simulink model "Simulation1"  (R2017b)
settings: Solver=FixedStepDiscrete  StartTime=0.0  StopTime=N/Fs  RelTol=1e-3
values from neighbouring files (symbols this model uses):
  A = 0.5*(nLev-1)    (= 0.5)    [Model3.m]
  ftest = 9e3    (= 9000)    [Model3.m]    (also in Model3_LTE.m = 2250)
  Ts = 1/Fs    (= 2.03450520833e-06)    [Model3.m]    (also in Model3_LTE.m = 1/Fs)
undefined symbols (not defined in the file or in its folder): a, b, c, g
libraries: dspsigops x16, simulink x8, dspsrcs4 x2
(part 1 of 3)
settings Model: Creator=o_cotte  LastModifiedBy=o_cotte

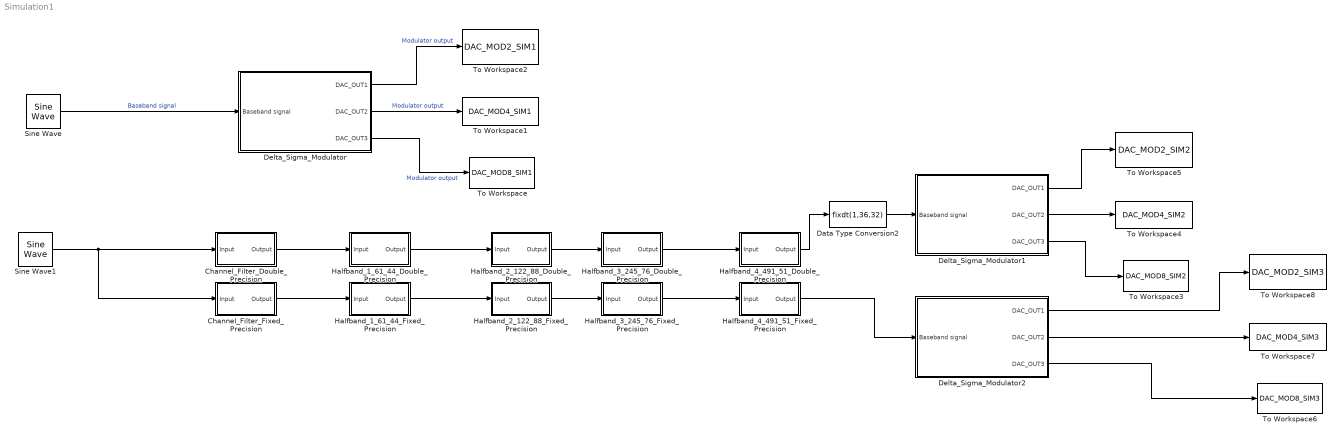
== system Simulation1 ==
  Channel_Filter_Double_Precision : Subsystem  Tag=FilterWizardSubSystem
      settings: ErrorFcn=dspFilterRealizedInBasicElemsAlgLoopErrFcnCallback
  Channel_Filter_Fixed_Precision : Subsystem  Tag=FilterWizardSubSystem
      settings: ErrorFcn=dspFilterRealizedInBasicElemsAlgLoopErrFcnCallback
  Data Type Conversion2 : DataTypeConversion  OutDataTypeStr=fixdt(1,36,32)  LockScale=on
  Delta_Sigma_Modulator : Subsystem
  Delta_Sigma_Modulator1 : Subsystem
  Delta_Sigma_Modulator2 : Subsystem
  Halfband_1_61_44_Double_Precision : Subsystem  Tag=FilterWizardSubSystem
      settings: ErrorFcn=dspFilterRealizedInBasicElemsAlgLoopErrFcnCallback
  Halfband_1_61_44_Fixed_Precision : Subsystem  Tag=FilterWizardSubSystem
      settings: ErrorFcn=dspFilterRealizedInBasicElemsAlgLoopErrFcnCallback
  Halfband_2_122_88_Double_Precision : Subsystem  Tag=FilterWizardSubSystem
      settings: ErrorFcn=dspFilterRealizedInBasicElemsAlgLoopErrFcnCallback
  Halfband_2_122_88_Fixed_Precision : Subsystem  Tag=FilterWizardSubSystem
      settings: ErrorFcn=dspFilterRealizedInBasicElemsAlgLoopErrFcnCallback
  Halfband_3_245_76_Double_Precision : Subsystem  Tag=FilterWizardSubSystem
      settings: ErrorFcn=dspFilterRealizedInBasicElemsAlgLoopErrFcnCallback
  Halfband_3_245_76_Fixed_Precision : Subsystem  Tag=FilterWizardSubSystem
      settings: ErrorFcn=dspFilterRealizedInBasicElemsAlgLoopErrFcnCallback
  Halfband_4_491_51_Double_Precision : Subsystem  Tag=FilterWizardSubSystem
      settings: ErrorFcn=dspFilterRealizedInBasicElemsAlgLoopErrFcnCallback
  Halfband_4_491_51_Fixed_Precision : Subsystem  Tag=FilterWizardSubSystem
      settings: ErrorFcn=dspFilterRealizedInBasicElemsAlgLoopErrFcnCallback
  Sine Wave : dspsrcs4/Sine Wave  Amplitude=0.77  Frequency=ftest  Phase=0  SampleMode=Discrete  OutComplex=Real  CompMethod=Trigonometric fcn  TableSize=Speed  SampleTime=Ts  SamplesPerFrame=1  ResetState=Restart at time zero  OutputFrames=on  dataType=double  wordLen=16  udDataType=sfix(16)  fracBitsMode=Best precision  numFracBits=15  OutDataTypeStr=double  LastOutDataTypeStr=double
  Sine Wave1 : dspsrcs4/Sine Wave  Amplitude=A  Frequency=ftest  Phase=0  SampleMode=Discrete  OutComplex=Real  CompMethod=Trigonometric fcn  TableSize=Speed  SampleTime=1/30.72e3  SamplesPerFrame=1  ResetState=Restart at time zero  OutputFrames=on  dataType=double  wordLen=16  udDataType=sfix(16)  fracBitsMode=Best precision  numFracBits=15  OutDataTypeStr=double  LastOutDataTypeStr=double
  To Workspace : ToWorkspace  VariableName=DAC_MOD8_SIM1  SampleTime=-1
  To Workspace1 : ToWorkspace  VariableName=DAC_MOD4_SIM1  SampleTime=-1
  To Workspace2 : ToWorkspace  VariableName=DAC_MOD2_SIM1  SampleTime=-1
  To Workspace3 : ToWorkspace  VariableName=DAC_MOD8_SIM2  SampleTime=-1
  To Workspace4 : ToWorkspace  VariableName=DAC_MOD4_SIM2  SampleTime=-1
  To Workspace5 : ToWorkspace  VariableName=DAC_MOD2_SIM2  SampleTime=-1
  To Workspace6 : ToWorkspace  VariableName=DAC_MOD8_SIM3  SampleTime=-1
  To Workspace7 : ToWorkspace  VariableName=DAC_MOD4_SIM3  SampleTime=-1
  To Workspace8 : ToWorkspace  VariableName=DAC_MOD2_SIM3  SampleTime=-1
  wires:
  Sine Wave/1 -> Delta_Sigma_Modulator/1(Baseband signal)  "Baseband signal"
  Delta_Sigma_Modulator/3(DAC_OUT3) -> To Workspace/1  "Modulator output"
  Delta_Sigma_Modulator/2(DAC_OUT2) -> To Workspace1/1  "Modulator output"
  Delta_Sigma_Modulator/1(DAC_OUT1) -> To Workspace2/1  "Modulator output"
  Channel_Filter_Double_Precision/1(Output) -> Halfband_1_61_44_Double_Precision/1(Input)
  Halfband_1_61_44_Double_Precision/1(Output) -> Halfband_2_122_88_Double_Precision/1(Input)
  Halfband_2_122_88_Double_Precision/1(Output) -> Halfband_3_245_76_Double_Precision/1(Input)
  Halfband_3_245_76_Double_Precision/1(Output) -> Halfband_4_491_51_Double_Precision/1(Input)
  Halfband_3_245_76_Fixed_Precision/1(Output) -> Halfband_4_491_51_Fixed_Precision/1(Input)
  Halfband_2_122_88_Fixed_Precision/1(Output) -> Halfband_3_245_76_Fixed_Precision/1(Input)
  Halfband_1_61_44_Fixed_Precision/1(Output) -> Halfband_2_122_88_Fixed_Precision/1(Input)
  Channel_Filter_Fixed_Precision/1(Output) -> Halfband_1_61_44_Fixed_Precision/1(Input)
  Sine Wave1/1 -> Channel_Filter_Fixed_Precision/1(Input), Channel_Filter_Double_Precision/1(Input)
  Halfband_4_491_51_Fixed_Precision/1(Output) -> Delta_Sigma_Modulator2/1(Baseband signal)
  Delta_Sigma_Modulator1/2(DAC_OUT2) -> To Workspace4/1
  Delta_Sigma_Modulator1/3(DAC_OUT3) -> To Workspace3/1
  Delta_Sigma_Modulator1/1(DAC_OUT1) -> To Workspace5/1
  Delta_Sigma_Modulator2/2(DAC_OUT2) -> To Workspace7/1
  Delta_Sigma_Modulator2/1(DAC_OUT1) -> To Workspace8/1
  Delta_Sigma_Modulator2/3(DAC_OUT3) -> To Workspace6/1
  Data Type Conversion2/1 -> Delta_Sigma_Modulator1/1(Baseband signal)
  Halfband_4_491_51_Double_Precision/1(Output) -> Data Type Conversion2/1

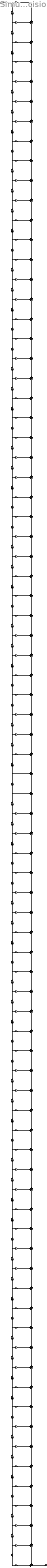
== system Simulation1/Channel_Filter_Double_Precision ==
  Input : Inport
  BodyDelay{2..80} (79 alike) : Delay  DelayLength=1  InitialCondition=0
  BodyLSum{2..80} (79 alike) : Sum  Inputs=++|  RndMeth=Nearest  SaturateOnIntegerOverflow=on  OutDataTypeStr=Inherit: Same as first input
  b(1) : Gain  Gain=0.00196720306212561482  ParamDataTypeStr=double  RndMeth=Nearest  SaturateOnIntegerOverflow=on  OutDataTypeStr=Inherit: Same as input
  b(10) : Gain  Gain=0.00124990544593627895  ParamDataTypeStr=double  RndMeth=Nearest  SaturateOnIntegerOverflow=on  OutDataTypeStr=Inherit: Same as input
  b(11) : Gain  Gain=0.00637795842127835896  ParamDataTypeStr=double  RndMeth=Nearest  SaturateOnIntegerOverflow=on  OutDataTypeStr=Inherit: Same as input
  b(12) : Gain  Gain=-0.00686348731071946636  ParamDataTypeStr=double  RndMeth=Nearest  SaturateOnIntegerOverflow=on  OutDataTypeStr=Inherit: Same as input
  b(13) : Gain  Gain=-0.00221497240802292442  ParamDataTypeStr=double  RndMeth=Nearest  SaturateOnIntegerOverflow=on  OutDataTypeStr=Inherit: Same as input
  b(14) : Gain  Gain=0.0103098487689475479  ParamDataTypeStr=double  RndMeth=Nearest  SaturateOnIntegerOverflow=on  OutDataTypeStr=Inherit: Same as input
  b(15) : Gain  Gain=-0.00579957522561930575  ParamDataTypeStr=double  RndMeth=Nearest  SaturateOnIntegerOverflow=on  OutDataTypeStr=Inherit: Same as input
  b(16) : Gain  Gain=-0.00783937474606764828  ParamDataTypeStr=double  RndMeth=Nearest  SaturateOnIntegerOverflow=on  OutDataTypeStr=Inherit: Same as input
  b(17) : Gain  Gain=0.0135158399775277549  ParamDataTypeStr=double  RndMeth=Nearest  SaturateOnIntegerOverflow=on  OutDataTypeStr=Inherit: Same as input
  b(18) : Gain  Gain=-0.00155602281125578911  ParamDataTypeStr=double  RndMeth=Nearest  SaturateOnIntegerOverflow=on  OutDataTypeStr=Inherit: Same as input
  b(19) : Gain  Gain=-0.0151258138642529176  ParamDataTypeStr=double  RndMeth=Nearest  SaturateOnIntegerOverflow=on  OutDataTypeStr=Inherit: Same as input
  b(2) : Gain  Gain=0.00149425216106443691  ParamDataTypeStr=double  RndMeth=Nearest  SaturateOnIntegerOverflow=on  OutDataTypeStr=Inherit: Same as input
  b(20) : Gain  Gain=0.0142568491821450007  ParamDataTypeStr=double  RndMeth=Nearest  SaturateOnIntegerOverflow=on  OutDataTypeStr=Inherit: Same as input
  b(21) : Gain  Gain=0.00665092392134642753  ParamDataTypeStr=double  RndMeth=Nearest  SaturateOnIntegerOverflow=on  OutDataTypeStr=Inherit: Same as input
  b(22) : Gain  Gain=-0.0226731257471077807  ParamDataTypeStr=double  RndMeth=Nearest  SaturateOnIntegerOverflow=on  OutDataTypeStr=Inherit: Same as input
  b(23) : Gain  Gain=0.0104679129061562917  ParamDataTypeStr=double  RndMeth=Nearest  SaturateOnIntegerOverflow=on  OutDataTypeStr=Inherit: Same as input
  b(24) : Gain  Gain=0.018904809782294061  ParamDataTypeStr=double  RndMeth=Nearest  SaturateOnIntegerOverflow=on  OutDataTypeStr=Inherit: Same as input
  b(25) : Gain  Gain=-0.0281519456111425509  ParamDataTypeStr=double  RndMeth=Nearest  SaturateOnIntegerOverflow=on  OutDataTypeStr=Inherit: Same as input
  b(26) : Gain  Gain=3.77195008409268937e-05  ParamDataTypeStr=double  RndMeth=Nearest  SaturateOnIntegerOverflow=on  OutDataTypeStr=Inherit: Same as input
  b(27) : Gain  Gain=0.0343690574379760388  ParamDataTypeStr=double  RndMeth=Nearest  SaturateOnIntegerOverflow=on  OutDataTypeStr=Inherit: Same as input
  b(28) : Gain  Gain=-0.0283201893723893684  ParamDataTypeStr=double  RndMeth=Nearest  SaturateOnIntegerOverflow=on  OutDataTypeStr=Inherit: Same as input
  b(29) : Gain  Gain=-0.0191525533345231584  ParamDataTypeStr=double  RndMeth=Nearest  SaturateOnIntegerOverflow=on  OutDataTypeStr=Inherit: Same as input
  b(3) : Gain  Gain=-0.00400293320810243911  ParamDataTypeStr=double  RndMeth=Nearest  SaturateOnIntegerOverflow=on  OutDataTypeStr=Inherit: Same as input
  b(30) : Gain  Gain=0.0512858826615412086  ParamDataTypeStr=double  RndMeth=Nearest  SaturateOnIntegerOverflow=on  OutDataTypeStr=Inherit: Same as input
  b(31) : Gain  Gain=-0.0186277130508248137  ParamDataTypeStr=double  RndMeth=Nearest  SaturateOnIntegerOverflow=on  OutDataTypeStr=Inherit: Same as input
  b(32) : Gain  Gain=-0.0502110306645960694  ParamDataTypeStr=double  RndMeth=Nearest  SaturateOnIntegerOverflow=on  OutDataTypeStr=Inherit: Same as input
  b(33) : Gain  Gain=0.0672661641118006554  ParamDataTypeStr=double  RndMeth=Nearest  SaturateOnIntegerOverflow=on  OutDataTypeStr=Inherit: Same as input
  b(34) : Gain  Gain=0.00945698178191303231  ParamDataTypeStr=double  RndMeth=Nearest  SaturateOnIntegerOverflow=on  OutDataTypeStr=Inherit: Same as input
  b(35) : Gain  Gain=-0.102591535984214791  ParamDataTypeStr=double  RndMeth=Nearest  SaturateOnIntegerOverflow=on  OutDataTypeStr=Inherit: Same as input
  b(36) : Gain  Gain=0.0797527182394069389  ParamDataTypeStr=double  RndMeth=Nearest  SaturateOnIntegerOverflow=on  OutDataTypeStr=Inherit: Same as input
  b(37) : Gain  Gain=0.0877414496207477579  ParamDataTypeStr=double  RndMeth=Nearest  SaturateOnIntegerOverflow=on  OutDataTypeStr=Inherit: Same as input
  b(38) : Gain  Gain=-0.237055871068311774  ParamDataTypeStr=double  RndMeth=Nearest  SaturateOnIntegerOverflow=on  OutDataTypeStr=Inherit: Same as input
  b(39) : Gain  Gain=0.0866069815926385905  ParamDataTypeStr=double  RndMeth=Nearest  SaturateOnIntegerOverflow=on  OutDataTypeStr=Inherit: Same as input
  b(4) : Gain  Gain=0.00390100375479263085  ParamDataTypeStr=double  RndMeth=Nearest  SaturateOnIntegerOverflow=on  OutDataTypeStr=Inherit: Same as input
  b(42) : Gain  Gain=0.0866069815926385905  ParamDataTypeStr=double  RndMeth=Nearest  SaturateOnIntegerOverflow=on  OutDataTypeStr=Inherit: Same as input
  b(43) : Gain  Gain=-0.237055871068311774  ParamDataTypeStr=double  RndMeth=Nearest  SaturateOnIntegerOverflow=on  OutDataTypeStr=Inherit: Same as input
  b(44) : Gain  Gain=0.0877414496207477579  ParamDataTypeStr=double  RndMeth=Nearest  SaturateOnIntegerOverflow=on  OutDataTypeStr=Inherit: Same as input
  b(45) : Gain  Gain=0.0797527182394069389  ParamDataTypeStr=double  RndMeth=Nearest  SaturateOnIntegerOverflow=on  OutDataTypeStr=Inherit: Same as input
  b(46) : Gain  Gain=-0.102591535984214791  ParamDataTypeStr=double  RndMeth=Nearest  SaturateOnIntegerOverflow=on  OutDataTypeStr=Inherit: Same as input
  b(47) : Gain  Gain=0.00945698178191303231  ParamDataTypeStr=double  RndMeth=Nearest  SaturateOnIntegerOverflow=on  OutDataTypeStr=Inherit: Same as input
  b(48) : Gain  Gain=0.0672661641118006554  ParamDataTypeStr=double  RndMeth=Nearest  SaturateOnIntegerOverflow=on  OutDataTypeStr=Inherit: Same as input
  b(49) : Gain  Gain=-0.0502110306645960694  ParamDataTypeStr=double  RndMeth=Nearest  SaturateOnIntegerOverflow=on  OutDataTypeStr=Inherit: Same as input
  b(5) : Gain  Gain=-2.89147778793418149e-07  ParamDataTypeStr=double  RndMeth=Nearest  SaturateOnIntegerOverflow=on  OutDataTypeStr=Inherit: Same as input
  b(50) : Gain  Gain=-0.0186277130508248137  ParamDataTypeStr=double  RndMeth=Nearest  SaturateOnIntegerOverflow=on  OutDataTypeStr=Inherit: Same as input
  b(51) : Gain  Gain=0.0512858826615412086  ParamDataTypeStr=double  RndMeth=Nearest  SaturateOnIntegerOverflow=on  OutDataTypeStr=Inherit: Same as input
  b(52) : Gain  Gain=-0.0191525533345231584  ParamDataTypeStr=double  RndMeth=Nearest  SaturateOnIntegerOverflow=on  OutDataTypeStr=Inherit: Same as input
  b(53) : Gain  Gain=-0.0283201893723893684  ParamDataTypeStr=double  RndMeth=Nearest  SaturateOnIntegerOverflow=on  OutDataTypeStr=Inherit: Same as input
  b(54) : Gain  Gain=0.0343690574379760388  ParamDataTypeStr=double  RndMeth=Nearest  SaturateOnIntegerOverflow=on  OutDataTypeStr=Inherit: Same as input
  b(55) : Gain  Gain=3.77195008409268937e-05  ParamDataTypeStr=double  RndMeth=Nearest  SaturateOnIntegerOverflow=on  OutDataTypeStr=Inherit: Same as input
  b(56) : Gain  Gain=-0.0281519456111425509  ParamDataTypeStr=double  RndMeth=Nearest  SaturateOnIntegerOverflow=on  OutDataTypeStr=Inherit: Same as input
  b(57) : Gain  Gain=0.018904809782294061  ParamDataTypeStr=double  RndMeth=Nearest  SaturateOnIntegerOverflow=on  OutDataTypeStr=Inherit: Same as input
  b(58) : Gain  Gain=0.0104679129061562917  ParamDataTypeStr=double  RndMeth=Nearest  SaturateOnIntegerOverflow=on  OutDataTypeStr=Inherit: Same as input
  b(59) : Gain  Gain=-0.0226731257471077807  ParamDataTypeStr=double  RndMeth=Nearest  SaturateOnIntegerOverflow=on  OutDataTypeStr=Inherit: Same as input
  b(6) : Gain  Gain=-0.00382987035567847927  ParamDataTypeStr=double  RndMeth=Nearest  SaturateOnIntegerOverflow=on  OutDataTypeStr=Inherit: Same as input
  b(60) : Gain  Gain=0.00665092392134642753  ParamDataTypeStr=double  RndMeth=Nearest  SaturateOnIntegerOverflow=on  OutDataTypeStr=Inherit: Same as input
  b(61) : Gain  Gain=0.0142568491821450007  ParamDataTypeStr=double  RndMeth=Nearest  SaturateOnIntegerOverflow=on  OutDataTypeStr=Inherit: Same as input
  b(62) : Gain  Gain=-0.0151258138642529176  ParamDataTypeStr=double  RndMeth=Nearest  SaturateOnIntegerOverflow=on  OutDataTypeStr=Inherit: Same as input
  b(63) : Gain  Gain=-0.00155602281125578911  ParamDataTypeStr=double  RndMeth=Nearest  SaturateOnIntegerOverflow=on  OutDataTypeStr=Inherit: Same as input
  b(64) : Gain  Gain=0.0135158399775277549  ParamDataTypeStr=double  RndMeth=Nearest  SaturateOnIntegerOverflow=on  OutDataTypeStr=Inherit: Same as input
  b(65) : Gain  Gain=-0.00783937474606764828  ParamDataTypeStr=double  RndMeth=Nearest  SaturateOnIntegerOverflow=on  OutDataTypeStr=Inherit: Same as input
  b(66) : Gain  Gain=-0.00579957522561930575  ParamDataTypeStr=double  RndMeth=Nearest  SaturateOnIntegerOverflow=on  OutDataTypeStr=Inherit: Same as input
  b(67) : Gain  Gain=0.0103098487689475479  ParamDataTypeStr=double  RndMeth=Nearest  SaturateOnIntegerOverflow=on  OutDataTypeStr=Inherit: Same as input
  b(68) : Gain  Gain=-0.00221497240802292442  ParamDataTypeStr=double  RndMeth=Nearest  SaturateOnIntegerOverflow=on  OutDataTypeStr=Inherit: Same as input
  b(69) : Gain  Gain=-0.00686348731071946636  ParamDataTypeStr=double  RndMeth=Nearest  SaturateOnIntegerOverflow=on  OutDataTypeStr=Inherit: Same as input
  b(7) : Gain  Gain=0.00259524746093026722  ParamDataTypeStr=double  RndMeth=Nearest  SaturateOnIntegerOverflow=on  OutDataTypeStr=Inherit: Same as input
  b(70) : Gain  Gain=0.00637795842127835896  ParamDataTypeStr=double  RndMeth=Nearest  SaturateOnIntegerOverflow=on  OutDataTypeStr=Inherit: Same as input
  b(71) : Gain  Gain=0.00124990544593627895  ParamDataTypeStr=double  RndMeth=Nearest  SaturateOnIntegerOverflow=on  OutDataTypeStr=Inherit: Same as input
  b(72) : Gain  Gain=-0.00593452115673513431  ParamDataTypeStr=double  RndMeth=Nearest  SaturateOnIntegerOverflow=on  OutDataTypeStr=Inherit: Same as input
  b(73) : Gain  Gain=0.00299398664123881825  ParamDataTypeStr=double  RndMeth=Nearest  SaturateOnIntegerOverflow=on  OutDataTypeStr=Inherit: Same as input
  b(74) : Gain  Gain=0.00259524746093026722  ParamDataTypeStr=double  RndMeth=Nearest  SaturateOnIntegerOverflow=on  OutDataTypeStr=Inherit: Same as input
  b(75) : Gain  Gain=-0.00382987035567847927  ParamDataTypeStr=double  RndMeth=Nearest  SaturateOnIntegerOverflow=on  OutDataTypeStr=Inherit: Same as input
  b(76) : Gain  Gain=-2.89147778793418149e-07  ParamDataTypeStr=double  RndMeth=Nearest  SaturateOnIntegerOverflow=on  OutDataTypeStr=Inherit: Same as input
  b(77) : Gain  Gain=0.00390100375479263085  ParamDataTypeStr=double  RndMeth=Nearest  SaturateOnIntegerOverflow=on  OutDataTypeStr=Inherit: Same as input
  b(78) : Gain  Gain=-0.00400293320810243911  ParamDataTypeStr=double  RndMeth=Nearest  SaturateOnIntegerOverflow=on  OutDataTypeStr=Inherit: Same as input
  b(79) : Gain  Gain=0.00149425216106443691  ParamDataTypeStr=double  RndMeth=Nearest  SaturateOnIntegerOverflow=on  OutDataTypeStr=Inherit: Same as input
  b(8) : Gain  Gain=0.00299398664123881825  ParamDataTypeStr=double  RndMeth=Nearest  SaturateOnIntegerOverflow=on  OutDataTypeStr=Inherit: Same as input
  b(80) : Gain  Gain=0.00196720306212561482  ParamDataTypeStr=double  RndMeth=Nearest  SaturateOnIntegerOverflow=on  OutDataTypeStr=Inherit: Same as input
  b(9) : Gain  Gain=-0.00593452115673513431  ParamDataTypeStr=double  RndMeth=Nearest  SaturateOnIntegerOverflow=on  OutDataTypeStr=Inherit: Same as input
  Output : Outport
  wires:
  Input/1 -> b(1)/1, BodyDelay2/1
  b(1)/1 -> BodyLSum2/2
  BodyDelay2/1 -> b(2)/1, BodyDelay3/1
  b(2)/1 -> BodyLSum2/1
  BodyLSum2/1 -> BodyLSum3/2
  BodyDelay3/1 -> b(3)/1, BodyDelay4/1
  b(3)/1 -> BodyLSum3/1
  BodyLSum3/1 -> BodyLSum4/2
  BodyDelay4/1 -> b(4)/1, BodyDelay5/1
  b(4)/1 -> BodyLSum4/1
  BodyLSum4/1 -> BodyLSum5/2
  BodyDelay5/1 -> b(5)/1, BodyDelay6/1
  b(5)/1 -> BodyLSum5/1
  BodyLSum5/1 -> BodyLSum6/2
  BodyDelay6/1 -> b(6)/1, BodyDelay7/1
  b(6)/1 -> BodyLSum6/1
  BodyLSum6/1 -> BodyLSum7/2
  BodyDelay7/1 -> b(7)/1, BodyDelay8/1
  b(7)/1 -> BodyLSum7/1
  BodyLSum7/1 -> BodyLSum8/2
  BodyDelay8/1 -> b(8)/1, BodyDelay9/1
  b(8)/1 -> BodyLSum8/1
  BodyLSum8/1 -> BodyLSum9/2
  BodyDelay9/1 -> b(9)/1, BodyDelay10/1
  b(9)/1 -> BodyLSum9/1
  BodyLSum9/1 -> BodyLSum10/2
  BodyDelay10/1 -> b(10)/1, BodyDelay11/1
  b(10)/1 -> BodyLSum10/1
  BodyLSum10/1 -> BodyLSum11/2
  BodyDelay11/1 -> b(11)/1, BodyDelay12/1
  b(11)/1 -> BodyLSum11/1
  BodyLSum11/1 -> BodyLSum12/2
  BodyDelay12/1 -> b(12)/1, BodyDelay13/1
  b(12)/1 -> BodyLSum12/1
  BodyLSum12/1 -> BodyLSum13/2
  BodyDelay13/1 -> b(13)/1, BodyDelay14/1
  b(13)/1 -> BodyLSum13/1
  BodyLSum13/1 -> BodyLSum14/2
  BodyDelay14/1 -> b(14)/1, BodyDelay15/1
  b(14)/1 -> BodyLSum14/1
  BodyLSum14/1 -> BodyLSum15/2
  BodyDelay15/1 -> b(15)/1, BodyDelay16/1
  b(15)/1 -> BodyLSum15/1
  BodyLSum15/1 -> BodyLSum16/2
  BodyDelay16/1 -> b(16)/1, BodyDelay17/1
  b(16)/1 -> BodyLSum16/1
  BodyLSum16/1 -> BodyLSum17/2
  BodyDelay17/1 -> b(17)/1, BodyDelay18/1
  b(17)/1 -> BodyLSum17/1
  BodyLSum17/1 -> BodyLSum18/2
  BodyDelay18/1 -> b(18)/1, BodyDelay19/1
  b(18)/1 -> BodyLSum18/1
  BodyLSum18/1 -> BodyLSum19/2
  BodyDelay19/1 -> b(19)/1, BodyDelay20/1
  b(19)/1 -> BodyLSum19/1
  BodyLSum19/1 -> BodyLSum20/2
  BodyDelay20/1 -> b(20)/1, BodyDelay21/1
  b(20)/1 -> BodyLSum20/1
  BodyLSum20/1 -> BodyLSum21/2
  BodyDelay21/1 -> b(21)/1, BodyDelay22/1
  b(21)/1 -> BodyLSum21/1
  BodyLSum21/1 -> BodyLSum22/2
  BodyDelay22/1 -> b(22)/1, BodyDelay23/1
  b(22)/1 -> BodyLSum22/1
  BodyLSum22/1 -> BodyLSum23/2
  BodyDelay23/1 -> b(23)/1, BodyDelay24/1
  b(23)/1 -> BodyLSum23/1
  BodyLSum23/1 -> BodyLSum24/2
  BodyDelay24/1 -> b(24)/1, BodyDelay25/1
  b(24)/1 -> BodyLSum24/1
  BodyLSum24/1 -> BodyLSum25/2
  BodyDelay25/1 -> b(25)/1, BodyDelay26/1
  b(25)/1 -> BodyLSum25/1
  BodyLSum25/1 -> BodyLSum26/2
  BodyDelay26/1 -> b(26)/1, BodyDelay27/1
  b(26)/1 -> BodyLSum26/1
  BodyLSum26/1 -> BodyLSum27/2
  BodyDelay27/1 -> b(27)/1, BodyDelay28/1
  b(27)/1 -> BodyLSum27/1
  BodyLSum27/1 -> BodyLSum28/2
  BodyDelay28/1 -> b(28)/1, BodyDelay29/1
  b(28)/1 -> BodyLSum28/1
  BodyLSum28/1 -> BodyLSum29/2
  BodyDelay29/1 -> b(29)/1, BodyDelay30/1
  b(29)/1 -> BodyLSum29/1
  BodyLSum29/1 -> BodyLSum30/2
  BodyDelay30/1 -> b(30)/1, BodyDelay31/1
  b(30)/1 -> BodyLSum30/1
  BodyLSum30/1 -> BodyLSum31/2
  BodyDelay31/1 -> b(31)/1, BodyDelay32/1
  b(31)/1 -> BodyLSum31/1
  BodyLSum31/1 -> BodyLSum32/2
  BodyDelay32/1 -> b(32)/1, BodyDelay33/1
  b(32)/1 -> BodyLSum32/1
  BodyLSum32/1 -> BodyLSum33/2
  BodyDelay33/1 -> b(33)/1, BodyDelay34/1
  b(33)/1 -> BodyLSum33/1
  BodyLSum33/1 -> BodyLSum34/2
  BodyDelay34/1 -> b(34)/1, BodyDelay35/1
  b(34)/1 -> BodyLSum34/1
  BodyLSum34/1 -> BodyLSum35/2
  BodyDelay35/1 -> b(35)/1, BodyDelay36/1
  b(35)/1 -> BodyLSum35/1
  BodyLSum35/1 -> BodyLSum36/2
  BodyDelay36/1 -> b(36)/1, BodyDelay37/1
  b(36)/1 -> BodyLSum36/1
  BodyLSum36/1 -> BodyLSum37/2
  BodyDelay37/1 -> b(37)/1, BodyDelay38/1
  b(37)/1 -> BodyLSum37/1
  BodyLSum37/1 -> BodyLSum38/2
  BodyDelay38/1 -> b(38)/1, BodyDelay39/1
  b(38)/1 -> BodyLSum38/1
  BodyLSum38/1 -> BodyLSum39/2
  BodyDelay39/1 -> b(39)/1, BodyDelay40/1
  b(39)/1 -> BodyLSum39/1
  BodyLSum39/1 -> BodyLSum40/2
  BodyDelay40/1 -> BodyLSum40/1, BodyDelay41/1
  BodyLSum40/1 -> BodyLSum41/2
  BodyDelay41/1 -> BodyLSum41/1, BodyDelay42/1
  BodyLSum41/1 -> BodyLSum42/2
  BodyDelay42/1 -> b(42)/1, BodyDelay43/1
  b(42)/1 -> BodyLSum42/1
  BodyLSum42/1 -> BodyLSum43/2
  BodyDelay43/1 -> b(43)/1, BodyDelay44/1
  b(43)/1 -> BodyLSum43/1
  BodyLSum43/1 -> BodyLSum44/2
  BodyDelay44/1 -> b(44)/1, BodyDelay45/1
  b(44)/1 -> BodyLSum44/1
  BodyLSum44/1 -> BodyLSum45/2
  BodyDelay45/1 -> b(45)/1, BodyDelay46/1
  b(45)/1 -> BodyLSum45/1
  BodyLSum45/1 -> BodyLSum46/2
  BodyDelay46/1 -> b(46)/1, BodyDelay47/1
  b(46)/1 -> BodyLSum46/1
  BodyLSum46/1 -> BodyLSum47/2
  BodyDelay47/1 -> b(47)/1, BodyDelay48/1
  b(47)/1 -> BodyLSum47/1
  BodyLSum47/1 -> BodyLSum48/2
  BodyDelay48/1 -> b(48)/1, BodyDelay49/1
  b(48)/1 -> BodyLSum48/1
  BodyLSum48/1 -> BodyLSum49/2
  BodyDelay49/1 -> b(49)/1, BodyDelay50/1
  b(49)/1 -> BodyLSum49/1
  BodyLSum49/1 -> BodyLSum50/2
  BodyDelay50/1 -> b(50)/1, BodyDelay51/1
  b(50)/1 -> BodyLSum50/1
  BodyLSum50/1 -> BodyLSum51/2
  BodyDelay51/1 -> b(51)/1, BodyDelay52/1
  b(51)/1 -> BodyLSum51/1
  BodyLSum51/1 -> BodyLSum52/2
  BodyDelay52/1 -> b(52)/1, BodyDelay53/1
  b(52)/1 -> BodyLSum52/1
  BodyLSum52/1 -> BodyLSum53/2
  BodyDelay53/1 -> b(53)/1, BodyDelay54/1
  b(53)/1 -> BodyLSum53/1
  BodyLSum53/1 -> BodyLSum54/2
  BodyDelay54/1 -> b(54)/1, BodyDelay55/1
  b(54)/1 -> BodyLSum54/1
  BodyLSum54/1 -> BodyLSum55/2
  BodyDelay55/1 -> b(55)/1, BodyDelay56/1
  b(55)/1 -> BodyLSum55/1
  BodyLSum55/1 -> BodyLSum56/2
  BodyDelay56/1 -> b(56)/1, BodyDelay57/1
  b(56)/1 -> BodyLSum56/1
  BodyLSum56/1 -> BodyLSum57/2
  BodyDelay57/1 -> b(57)/1, BodyDelay58/1
  b(57)/1 -> BodyLSum57/1
  BodyLSum57/1 -> BodyLSum58/2
  BodyDelay58/1 -> b(58)/1, BodyDelay59/1
  b(58)/1 -> BodyLSum58/1
  BodyLSum58/1 -> BodyLSum59/2
  BodyDelay59/1 -> b(59)/1, BodyDelay60/1
  b(59)/1 -> BodyLSum59/1
  BodyLSum59/1 -> BodyLSum60/2
  BodyDelay60/1 -> b(60)/1, BodyDelay61/1
  b(60)/1 -> BodyLSum60/1
  BodyLSum60/1 -> BodyLSum61/2
  BodyDelay61/1 -> b(61)/1, BodyDelay62/1
  b(61)/1 -> BodyLSum61/1
  BodyLSum61/1 -> BodyLSum62/2
  BodyDelay62/1 -> b(62)/1, BodyDelay63/1
  b(62)/1 -> BodyLSum62/1
  BodyLSum62/1 -> BodyLSum63/2
  BodyDelay63/1 -> b(63)/1, BodyDelay64/1
  b(63)/1 -> BodyLSum63/1
  BodyLSum63/1 -> BodyLSum64/2
  BodyDelay64/1 -> b(64)/1, BodyDelay65/1
  b(64)/1 -> BodyLSum64/1
  BodyLSum64/1 -> BodyLSum65/2
  BodyDelay65/1 -> b(65)/1, BodyDelay66/1
  b(65)/1 -> BodyLSum65/1
  BodyLSum65/1 -> BodyLSum66/2
  BodyDelay66/1 -> b(66)/1, BodyDelay67/1
  b(66)/1 -> BodyLSum66/1
  BodyLSum66/1 -> BodyLSum67/2
  BodyDelay67/1 -> b(67)/1, BodyDelay68/1
  b(67)/1 -> BodyLSum67/1
  BodyLSum67/1 -> BodyLSum68/2
  BodyDelay68/1 -> b(68)/1, BodyDelay69/1
  b(68)/1 -> BodyLSum68/1
  BodyLSum68/1 -> BodyLSum69/2
  BodyDelay69/1 -> b(69)/1, BodyDelay70/1
  b(69)/1 -> BodyLSum69/1
  BodyLSum69/1 -> BodyLSum70/2
  BodyDelay70/1 -> b(70)/1, BodyDelay71/1
  b(70)/1 -> BodyLSum70/1
  BodyLSum70/1 -> BodyLSum71/2
  BodyDelay71/1 -> b(71)/1, BodyDelay72/1
  b(71)/1 -> BodyLSum71/1
  BodyLSum71/1 -> BodyLSum72/2
  BodyDelay72/1 -> b(72)/1, BodyDelay73/1
  b(72)/1 -> BodyLSum72/1
  BodyLSum72/1 -> BodyLSum73/2
  BodyDelay73/1 -> b(73)/1, BodyDelay74/1
  b(73)/1 -> BodyLSum73/1
  BodyLSum73/1 -> BodyLSum74/2
  BodyDelay74/1 -> b(74)/1, BodyDelay75/1
  b(74)/1 -> BodyLSum74/1
  BodyLSum74/1 -> BodyLSum75/2
  BodyDelay75/1 -> b(75)/1, BodyDelay76/1
  b(75)/1 -> BodyLSum75/1
  BodyLSum75/1 -> BodyLSum76/2
  BodyDelay76/1 -> b(76)/1, BodyDelay77/1
  b(76)/1 -> BodyLSum76/1
  BodyLSum76/1 -> BodyLSum77/2
  BodyDelay77/1 -> b(77)/1, BodyDelay78/1
  b(77)/1 -> BodyLSum77/1
  BodyLSum77/1 -> BodyLSum78/2
  BodyDelay78/1 -> b(78)/1, BodyDelay79/1
  b(78)/1 -> BodyLSum78/1
  BodyLSum78/1 -> BodyLSum79/2
  BodyDelay79/1 -> b(79)/1, BodyDelay80/1
  b(79)/1 -> BodyLSum79/1
  BodyLSum79/1 -> BodyLSum80/1
  BodyDelay80/1 -> b(80)/1
  b(80)/1 -> BodyLSum80/2
  BodyLSum80/1 -> Output/1

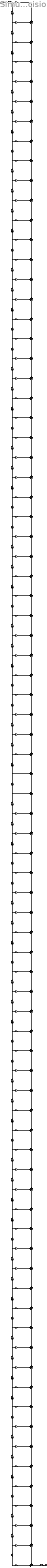
== system Simulation1/Channel_Filter_Fixed_Precision ==
  Input : Inport
  BodyDelay{2..80} (79 alike) : Delay  DelayLength=1  InitialCondition=0
  BodyLSum{2..80} (79 alike) : Sum  Inputs=++|  AccumDataTypeStr=fixdt(1,71,66)  OutDataTypeStr=fixdt(1,36,32)  SaturateOnIntegerOverflow=on
  ConvertIn : DataTypeConversion  OutDataTypeStr=fixdt(1,34,32)  RndMeth=Nearest  SaturateOnIntegerOverflow=on
  ConvertOut : DataTypeConversion  OutDataTypeStr=fixdt(1,34,30)  SaturateOnIntegerOverflow=on
  b(1) : Gain  Gain=0.00196720306212561482  ParamDataTypeStr=fixdt(1,36,34)  OutDataTypeStr=fixdt(1,36,32)  SaturateOnIntegerOverflow=on
  b(10) : Gain  Gain=0.00124990544593627895  ParamDataTypeStr=fixdt(1,36,34)  OutDataTypeStr=fixdt(1,36,32)  SaturateOnIntegerOverflow=on
  b(11) : Gain  Gain=0.00637795842127835896  ParamDataTypeStr=fixdt(1,36,34)  OutDataTypeStr=fixdt(1,36,32)  SaturateOnIntegerOverflow=on
  b(12) : Gain  Gain=-0.00686348731071946636  ParamDataTypeStr=fixdt(1,36,34)  OutDataTypeStr=fixdt(1,36,32)  SaturateOnIntegerOverflow=on
  b(13) : Gain  Gain=-0.00221497240802292442  ParamDataTypeStr=fixdt(1,36,34)  OutDataTypeStr=fixdt(1,36,32)  SaturateOnIntegerOverflow=on
  b(14) : Gain  Gain=0.0103098487689475479  ParamDataTypeStr=fixdt(1,36,34)  OutDataTypeStr=fixdt(1,36,32)  SaturateOnIntegerOverflow=on
  b(15) : Gain  Gain=-0.00579957522561930575  ParamDataTypeStr=fixdt(1,36,34)  OutDataTypeStr=fixdt(1,36,32)  SaturateOnIntegerOverflow=on
  b(16) : Gain  Gain=-0.00783937474606764828  ParamDataTypeStr=fixdt(1,36,34)  OutDataTypeStr=fixdt(1,36,32)  SaturateOnIntegerOverflow=on
  b(17) : Gain  Gain=0.0135158399775277549  ParamDataTypeStr=fixdt(1,36,34)  OutDataTypeStr=fixdt(1,36,32)  SaturateOnIntegerOverflow=on
  b(18) : Gain  Gain=-0.00155602281125578911  ParamDataTypeStr=fixdt(1,36,34)  OutDataTypeStr=fixdt(1,36,32)  SaturateOnIntegerOverflow=on
  b(19) : Gain  Gain=-0.0151258138642529176  ParamDataTypeStr=fixdt(1,36,34)  OutDataTypeStr=fixdt(1,36,32)  SaturateOnIntegerOverflow=on
  b(2) : Gain  Gain=0.00149425216106443691  ParamDataTypeStr=fixdt(1,36,34)  OutDataTypeStr=fixdt(1,36,32)  SaturateOnIntegerOverflow=on
  b(20) : Gain  Gain=0.0142568491821450007  ParamDataTypeStr=fixdt(1,36,34)  OutDataTypeStr=fixdt(1,36,32)  SaturateOnIntegerOverflow=on
  b(21) : Gain  Gain=0.00665092392134642753  ParamDataTypeStr=fixdt(1,36,34)  OutDataTypeStr=fixdt(1,36,32)  SaturateOnIntegerOverflow=on
  b(22) : Gain  Gain=-0.0226731257471077807  ParamDataTypeStr=fixdt(1,36,34)  OutDataTypeStr=fixdt(1,36,32)  SaturateOnIntegerOverflow=on
  b(23) : Gain  Gain=0.0104679129061562917  ParamDataTypeStr=fixdt(1,36,34)  OutDataTypeStr=fixdt(1,36,32)  SaturateOnIntegerOverflow=on
  b(24) : Gain  Gain=0.018904809782294061  ParamDataTypeStr=fixdt(1,36,34)  OutDataTypeStr=fixdt(1,36,32)  SaturateOnIntegerOverflow=on
  b(25) : Gain  Gain=-0.0281519456111425509  ParamDataTypeStr=fixdt(1,36,34)  OutDataTypeStr=fixdt(1,36,32)  SaturateOnIntegerOverflow=on
  b(26) : Gain  Gain=3.77195008409268937e-05  ParamDataTypeStr=fixdt(1,36,34)  OutDataTypeStr=fixdt(1,36,32)  SaturateOnIntegerOverflow=on
  b(27) : Gain  Gain=0.0343690574379760388  ParamDataTypeStr=fixdt(1,36,34)  OutDataTypeStr=fixdt(1,36,32)  SaturateOnIntegerOverflow=on
  b(28) : Gain  Gain=-0.0283201893723893684  ParamDataTypeStr=fixdt(1,36,34)  OutDataTypeStr=fixdt(1,36,32)  SaturateOnIntegerOverflow=on
  b(29) : Gain  Gain=-0.0191525533345231584  ParamDataTypeStr=fixdt(1,36,34)  OutDataTypeStr=fixdt(1,36,32)  SaturateOnIntegerOverflow=on
  b(3) : Gain  Gain=-0.00400293320810243911  ParamDataTypeStr=fixdt(1,36,34)  OutDataTypeStr=fixdt(1,36,32)  SaturateOnIntegerOverflow=on
  b(30) : Gain  Gain=0.0512858826615412086  ParamDataTypeStr=fixdt(1,36,34)  OutDataTypeStr=fixdt(1,36,32)  SaturateOnIntegerOverflow=on
  b(31) : Gain  Gain=-0.0186277130508248137  ParamDataTypeStr=fixdt(1,36,34)  OutDataTypeStr=fixdt(1,36,32)  SaturateOnIntegerOverflow=on
  b(32) : Gain  Gain=-0.0502110306645960694  ParamDataTypeStr=fixdt(1,36,34)  OutDataTypeStr=fixdt(1,36,32)  SaturateOnIntegerOverflow=on
  b(33) : Gain  Gain=0.0672661641118006554  ParamDataTypeStr=fixdt(1,36,34)  OutDataTypeStr=fixdt(1,36,32)  SaturateOnIntegerOverflow=on
  b(34) : Gain  Gain=0.00945698178191303231  ParamDataTypeStr=fixdt(1,36,34)  OutDataTypeStr=fixdt(1,36,32)  SaturateOnIntegerOverflow=on
  b(35) : Gain  Gain=-0.102591535984214791  ParamDataTypeStr=fixdt(1,36,34)  OutDataTypeStr=fixdt(1,36,32)  SaturateOnIntegerOverflow=on
  b(36) : Gain  Gain=0.0797527182394069389  ParamDataTypeStr=fixdt(1,36,34)  OutDataTypeStr=fixdt(1,36,32)  SaturateOnIntegerOverflow=on
  b(37) : Gain  Gain=0.0877414496207477579  ParamDataTypeStr=fixdt(1,36,34)  OutDataTypeStr=fixdt(1,36,32)  SaturateOnIntegerOverflow=on
  b(38) : Gain  Gain=-0.237055871068311774  ParamDataTypeStr=fixdt(1,36,34)  OutDataTypeStr=fixdt(1,36,32)  SaturateOnIntegerOverflow=on
  b(39) : Gain  Gain=0.0866069815926385905  ParamDataTypeStr=fixdt(1,36,34)  OutDataTypeStr=fixdt(1,36,32)  SaturateOnIntegerOverflow=on
  b(4) : Gain  Gain=0.00390100375479263085  ParamDataTypeStr=fixdt(1,36,34)  OutDataTypeStr=fixdt(1,36,32)  SaturateOnIntegerOverflow=on
  b(42) : Gain  Gain=0.0866069815926385905  ParamDataTypeStr=fixdt(1,36,34)  OutDataTypeStr=fixdt(1,36,32)  SaturateOnIntegerOverflow=on
  b(43) : Gain  Gain=-0.237055871068311774  ParamDataTypeStr=fixdt(1,36,34)  OutDataTypeStr=fixdt(1,36,32)  SaturateOnIntegerOverflow=on
  b(44) : Gain  Gain=0.0877414496207477579  ParamDataTypeStr=fixdt(1,36,34)  OutDataTypeStr=fixdt(1,36,32)  SaturateOnIntegerOverflow=on
  b(45) : Gain  Gain=0.0797527182394069389  ParamDataTypeStr=fixdt(1,36,34)  OutDataTypeStr=fixdt(1,36,32)  SaturateOnIntegerOverflow=on
  b(46) : Gain  Gain=-0.102591535984214791  ParamDataTypeStr=fixdt(1,36,34)  OutDataTypeStr=fixdt(1,36,32)  SaturateOnIntegerOverflow=on
  b(47) : Gain  Gain=0.00945698178191303231  ParamDataTypeStr=fixdt(1,36,34)  OutDataTypeStr=fixdt(1,36,32)  SaturateOnIntegerOverflow=on
  b(48) : Gain  Gain=0.0672661641118006554  ParamDataTypeStr=fixdt(1,36,34)  OutDataTypeStr=fixdt(1,36,32)  SaturateOnIntegerOverflow=on
  b(49) : Gain  Gain=-0.0502110306645960694  ParamDataTypeStr=fixdt(1,36,34)  OutDataTypeStr=fixdt(1,36,32)  SaturateOnIntegerOverflow=on
  b(5) : Gain  Gain=-2.89147778793418149e-07  ParamDataTypeStr=fixdt(1,36,34)  OutDataTypeStr=fixdt(1,36,32)  SaturateOnIntegerOverflow=on
  b(50) : Gain  Gain=-0.0186277130508248137  ParamDataTypeStr=fixdt(1,36,34)  OutDataTypeStr=fixdt(1,36,32)  SaturateOnIntegerOverflow=on
  b(51) : Gain  Gain=0.0512858826615412086  ParamDataTypeStr=fixdt(1,36,34)  OutDataTypeStr=fixdt(1,36,32)  SaturateOnIntegerOverflow=on
  b(52) : Gain  Gain=-0.0191525533345231584  ParamDataTypeStr=fixdt(1,36,34)  OutDataTypeStr=fixdt(1,36,32)  SaturateOnIntegerOverflow=on
  b(53) : Gain  Gain=-0.0283201893723893684  ParamDataTypeStr=fixdt(1,36,34)  OutDataTypeStr=fixdt(1,36,32)  SaturateOnIntegerOverflow=on
  b(54) : Gain  Gain=0.0343690574379760388  ParamDataTypeStr=fixdt(1,36,34)  OutDataTypeStr=fixdt(1,36,32)  SaturateOnIntegerOverflow=on
  b(55) : Gain  Gain=3.77195008409268937e-05  ParamDataTypeStr=fixdt(1,36,34)  OutDataTypeStr=fixdt(1,36,32)  SaturateOnIntegerOverflow=on
  b(56) : Gain  Gain=-0.0281519456111425509  ParamDataTypeStr=fixdt(1,36,34)  OutDataTypeStr=fixdt(1,36,32)  SaturateOnIntegerOverflow=on
  b(57) : Gain  Gain=0.018904809782294061  ParamDataTypeStr=fixdt(1,36,34)  OutDataTypeStr=fixdt(1,36,32)  SaturateOnIntegerOverflow=on
  b(58) : Gain  Gain=0.0104679129061562917  ParamDataTypeStr=fixdt(1,36,34)  OutDataTypeStr=fixdt(1,36,32)  SaturateOnIntegerOverflow=on
  b(59) : Gain  Gain=-0.0226731257471077807  ParamDataTypeStr=fixdt(1,36,34)  OutDataTypeStr=fixdt(1,36,32)  SaturateOnIntegerOverflow=on
  b(6) : Gain  Gain=-0.00382987035567847927  ParamDataTypeStr=fixdt(1,36,34)  OutDataTypeStr=fixdt(1,36,32)  SaturateOnIntegerOverflow=on
  b(60) : Gain  Gain=0.00665092392134642753  ParamDataTypeStr=fixdt(1,36,34)  OutDataTypeStr=fixdt(1,36,32)  SaturateOnIntegerOverflow=on
  b(61) : Gain  Gain=0.0142568491821450007  ParamDataTypeStr=fixdt(1,36,34)  OutDataTypeStr=fixdt(1,36,32)  SaturateOnIntegerOverflow=on
  b(62) : Gain  Gain=-0.0151258138642529176  ParamDataTypeStr=fixdt(1,36,34)  OutDataTypeStr=fixdt(1,36,32)  SaturateOnIntegerOverflow=on
  b(63) : Gain  Gain=-0.00155602281125578911  ParamDataTypeStr=fixdt(1,36,34)  OutDataTypeStr=fixdt(1,36,32)  SaturateOnIntegerOverflow=on
  b(64) : Gain  Gain=0.0135158399775277549  ParamDataTypeStr=fixdt(1,36,34)  OutDataTypeStr=fixdt(1,36,32)  SaturateOnIntegerOverflow=on
  b(65) : Gain  Gain=-0.00783937474606764828  ParamDataTypeStr=fixdt(1,36,34)  OutDataTypeStr=fixdt(1,36,32)  SaturateOnIntegerOverflow=on
  b(66) : Gain  Gain=-0.00579957522561930575  ParamDataTypeStr=fixdt(1,36,34)  OutDataTypeStr=fixdt(1,36,32)  SaturateOnIntegerOverflow=on
  b(67) : Gain  Gain=0.0103098487689475479  ParamDataTypeStr=fixdt(1,36,34)  OutDataTypeStr=fixdt(1,36,32)  SaturateOnIntegerOverflow=on
  b(68) : Gain  Gain=-0.00221497240802292442  ParamDataTypeStr=fixdt(1,36,34)  OutDataTypeStr=fixdt(1,36,32)  SaturateOnIntegerOverflow=on
  b(69) : Gain  Gain=-0.00686348731071946636  ParamDataTypeStr=fixdt(1,36,34)  OutDataTypeStr=fixdt(1,36,32)  SaturateOnIntegerOverflow=on
  b(7) : Gain  Gain=0.00259524746093026722  ParamDataTypeStr=fixdt(1,36,34)  OutDataTypeStr=fixdt(1,36,32)  SaturateOnIntegerOverflow=on
  b(70) : Gain  Gain=0.00637795842127835896  ParamDataTypeStr=fixdt(1,36,34)  OutDataTypeStr=fixdt(1,36,32)  SaturateOnIntegerOverflow=on
  b(71) : Gain  Gain=0.00124990544593627895  ParamDataTypeStr=fixdt(1,36,34)  OutDataTypeStr=fixdt(1,36,32)  SaturateOnIntegerOverflow=on
  b(72) : Gain  Gain=-0.00593452115673513431  ParamDataTypeStr=fixdt(1,36,34)  OutDataTypeStr=fixdt(1,36,32)  SaturateOnIntegerOverflow=on
  b(73) : Gain  Gain=0.00299398664123881825  ParamDataTypeStr=fixdt(1,36,34)  OutDataTypeStr=fixdt(1,36,32)  SaturateOnIntegerOverflow=on
  b(74) : Gain  Gain=0.00259524746093026722  ParamDataTypeStr=fixdt(1,36,34)  OutDataTypeStr=fixdt(1,36,32)  SaturateOnIntegerOverflow=on
  b(75) : Gain  Gain=-0.00382987035567847927  ParamDataTypeStr=fixdt(1,36,34)  OutDataTypeStr=fixdt(1,36,32)  SaturateOnIntegerOverflow=on
  b(76) : Gain  Gain=-2.89147778793418149e-07  ParamDataTypeStr=fixdt(1,36,34)  OutDataTypeStr=fixdt(1,36,32)  SaturateOnIntegerOverflow=on
  b(77) : Gain  Gain=0.00390100375479263085  ParamDataTypeStr=fixdt(1,36,34)  OutDataTypeStr=fixdt(1,36,32)  SaturateOnIntegerOverflow=on
  b(78) : Gain  Gain=-0.00400293320810243911  ParamDataTypeStr=fixdt(1,36,34)  OutDataTypeStr=fixdt(1,36,32)  SaturateOnIntegerOverflow=on
  b(79) : Gain  Gain=0.00149425216106443691  ParamDataTypeStr=fixdt(1,36,34)  OutDataTypeStr=fixdt(1,36,32)  SaturateOnIntegerOverflow=on
  b(8) : Gain  Gain=0.00299398664123881825  ParamDataTypeStr=fixdt(1,36,34)  OutDataTypeStr=fixdt(1,36,32)  SaturateOnIntegerOverflow=on
  b(80) : Gain  Gain=0.00196720306212561482  ParamDataTypeStr=fixdt(1,36,34)  OutDataTypeStr=fixdt(1,36,32)  SaturateOnIntegerOverflow=on
  b(9) : Gain  Gain=-0.00593452115673513431  ParamDataTypeStr=fixdt(1,36,34)  OutDataTypeStr=fixdt(1,36,32)  SaturateOnIntegerOverflow=on
  Output : Outport
  wires:
  Input/1 -> ConvertIn/1
  b(1)/1 -> BodyLSum2/2
  ConvertIn/1 -> b(1)/1, BodyDelay2/1
  BodyDelay2/1 -> b(2)/1, BodyDelay3/1
  b(2)/1 -> BodyLSum2/1
  BodyLSum2/1 -> BodyLSum3/2
  BodyDelay3/1 -> b(3)/1, BodyDelay4/1
  b(3)/1 -> BodyLSum3/1
  BodyLSum3/1 -> BodyLSum4/2
  BodyDelay4/1 -> b(4)/1, BodyDelay5/1
  b(4)/1 -> BodyLSum4/1
  BodyLSum4/1 -> BodyLSum5/2
  BodyDelay5/1 -> b(5)/1, BodyDelay6/1
  b(5)/1 -> BodyLSum5/1
  BodyLSum5/1 -> BodyLSum6/2
  BodyDelay6/1 -> b(6)/1, BodyDelay7/1
  b(6)/1 -> BodyLSum6/1
  BodyLSum6/1 -> BodyLSum7/2
  BodyDelay7/1 -> b(7)/1, BodyDelay8/1
  b(7)/1 -> BodyLSum7/1
  BodyLSum7/1 -> BodyLSum8/2
  BodyDelay8/1 -> b(8)/1, BodyDelay9/1
  b(8)/1 -> BodyLSum8/1
  BodyLSum8/1 -> BodyLSum9/2
  BodyDelay9/1 -> b(9)/1, BodyDelay10/1
  b(9)/1 -> BodyLSum9/1
  BodyLSum9/1 -> BodyLSum10/2
  BodyDelay10/1 -> b(10)/1, BodyDelay11/1
  b(10)/1 -> BodyLSum10/1
  BodyLSum10/1 -> BodyLSum11/2
  BodyDelay11/1 -> b(11)/1, BodyDelay12/1
  b(11)/1 -> BodyLSum11/1
  BodyLSum11/1 -> BodyLSum12/2
  BodyDelay12/1 -> b(12)/1, BodyDelay13/1
  b(12)/1 -> BodyLSum12/1
  BodyLSum12/1 -> BodyLSum13/2
  BodyDelay13/1 -> b(13)/1, BodyDelay14/1
  b(13)/1 -> BodyLSum13/1
  BodyLSum13/1 -> BodyLSum14/2
  BodyDelay14/1 -> b(14)/1, BodyDelay15/1
  b(14)/1 -> BodyLSum14/1
  BodyLSum14/1 -> BodyLSum15/2
  BodyDelay15/1 -> b(15)/1, BodyDelay16/1
  b(15)/1 -> BodyLSum15/1
  BodyLSum15/1 -> BodyLSum16/2
  BodyDelay16/1 -> b(16)/1, BodyDelay17/1
  b(16)/1 -> BodyLSum16/1
  BodyLSum16/1 -> BodyLSum17/2
  BodyDelay17/1 -> b(17)/1, BodyDelay18/1
  b(17)/1 -> BodyLSum17/1
  BodyLSum17/1 -> BodyLSum18/2
  BodyDelay18/1 -> b(18)/1, BodyDelay19/1
  b(18)/1 -> BodyLSum18/1
  BodyLSum18/1 -> BodyLSum19/2
  BodyDelay19/1 -> b(19)/1, BodyDelay20/1
  b(19)/1 -> BodyLSum19/1
  BodyLSum19/1 -> BodyLSum20/2
  BodyDelay20/1 -> b(20)/1, BodyDelay21/1
  b(20)/1 -> BodyLSum20/1
  BodyLSum20/1 -> BodyLSum21/2
  BodyDelay21/1 -> b(21)/1, BodyDelay22/1
  b(21)/1 -> BodyLSum21/1
  BodyLSum21/1 -> BodyLSum22/2
  BodyDelay22/1 -> b(22)/1, BodyDelay23/1
  b(22)/1 -> BodyLSum22/1
  BodyLSum22/1 -> BodyLSum23/2
  BodyDelay23/1 -> b(23)/1, BodyDelay24/1
  b(23)/1 -> BodyLSum23/1
  BodyLSum23/1 -> BodyLSum24/2
  BodyDelay24/1 -> b(24)/1, BodyDelay25/1
  b(24)/1 -> BodyLSum24/1
  BodyLSum24/1 -> BodyLSum25/2
  BodyDelay25/1 -> b(25)/1, BodyDelay26/1
  b(25)/1 -> BodyLSum25/1
  BodyLSum25/1 -> BodyLSum26/2
  BodyDelay26/1 -> b(26)/1, BodyDelay27/1
  b(26)/1 -> BodyLSum26/1
  BodyLSum26/1 -> BodyLSum27/2
  BodyDelay27/1 -> b(27)/1, BodyDelay28/1
  b(27)/1 -> BodyLSum27/1
  BodyLSum27/1 -> BodyLSum28/2
  BodyDelay28/1 -> b(28)/1, BodyDelay29/1
  b(28)/1 -> BodyLSum28/1
  BodyLSum28/1 -> BodyLSum29/2
  BodyDelay29/1 -> b(29)/1, BodyDelay30/1
  b(29)/1 -> BodyLSum29/1
  BodyLSum29/1 -> BodyLSum30/2
  BodyDelay30/1 -> b(30)/1, BodyDelay31/1
  b(30)/1 -> BodyLSum30/1
  BodyLSum30/1 -> BodyLSum31/2
  BodyDelay31/1 -> b(31)/1, BodyDelay32/1
  b(31)/1 -> BodyLSum31/1
  BodyLSum31/1 -> BodyLSum32/2
  BodyDelay32/1 -> b(32)/1, BodyDelay33/1
  b(32)/1 -> BodyLSum32/1
  BodyLSum32/1 -> BodyLSum33/2
  BodyDelay33/1 -> b(33)/1, BodyDelay34/1
  b(33)/1 -> BodyLSum33/1
  BodyLSum33/1 -> BodyLSum34/2
  BodyDelay34/1 -> b(34)/1, BodyDelay35/1
  b(34)/1 -> BodyLSum34/1
  BodyLSum34/1 -> BodyLSum35/2
  BodyDelay35/1 -> b(35)/1, BodyDelay36/1
  b(35)/1 -> BodyLSum35/1
  BodyLSum35/1 -> BodyLSum36/2
  BodyDelay36/1 -> b(36)/1, BodyDelay37/1
  b(36)/1 -> BodyLSum36/1
  BodyLSum36/1 -> BodyLSum37/2
  BodyDelay37/1 -> b(37)/1, BodyDelay38/1
  b(37)/1 -> BodyLSum37/1
  BodyLSum37/1 -> BodyLSum38/2
  BodyDelay38/1 -> b(38)/1, BodyDelay39/1
  b(38)/1 -> BodyLSum38/1
  BodyLSum38/1 -> BodyLSum39/2
  BodyDelay39/1 -> b(39)/1, BodyDelay40/1
  b(39)/1 -> BodyLSum39/1
  BodyLSum39/1 -> BodyLSum40/2
  BodyDelay40/1 -> BodyLSum40/1, BodyDelay41/1
  BodyLSum40/1 -> BodyLSum41/2
  BodyDelay41/1 -> BodyLSum41/1, BodyDelay42/1
  BodyLSum41/1 -> BodyLSum42/2
  BodyDelay42/1 -> b(42)/1, BodyDelay43/1
  b(42)/1 -> BodyLSum42/1
  BodyLSum42/1 -> BodyLSum43/2
  BodyDelay43/1 -> b(43)/1, BodyDelay44/1
  b(43)/1 -> BodyLSum43/1
  BodyLSum43/1 -> BodyLSum44/2
  BodyDelay44/1 -> b(44)/1, BodyDelay45/1
  b(44)/1 -> BodyLSum44/1
  BodyLSum44/1 -> BodyLSum45/2
  BodyDelay45/1 -> b(45)/1, BodyDelay46/1
  b(45)/1 -> BodyLSum45/1
  BodyLSum45/1 -> BodyLSum46/2
  BodyDelay46/1 -> b(46)/1, BodyDelay47/1
  b(46)/1 -> BodyLSum46/1
  BodyLSum46/1 -> BodyLSum47/2
  BodyDelay47/1 -> b(47)/1, BodyDelay48/1
  b(47)/1 -> BodyLSum47/1
  BodyLSum47/1 -> BodyLSum48/2
  BodyDelay48/1 -> b(48)/1, BodyDelay49/1
  b(48)/1 -> BodyLSum48/1
  BodyLSum48/1 -> BodyLSum49/2
  BodyDelay49/1 -> b(49)/1, BodyDelay50/1
  b(49)/1 -> BodyLSum49/1
  BodyLSum49/1 -> BodyLSum50/2
  BodyDelay50/1 -> b(50)/1, BodyDelay51/1
  b(50)/1 -> BodyLSum50/1
  BodyLSum50/1 -> BodyLSum51/2
  BodyDelay51/1 -> b(51)/1, BodyDelay52/1
  b(51)/1 -> BodyLSum51/1
  BodyLSum51/1 -> BodyLSum52/2
  BodyDelay52/1 -> b(52)/1, BodyDelay53/1
  b(52)/1 -> BodyLSum52/1
  BodyLSum52/1 -> BodyLSum53/2
  BodyDelay53/1 -> b(53)/1, BodyDelay54/1
  b(53)/1 -> BodyLSum53/1
  BodyLSum53/1 -> BodyLSum54/2
  BodyDelay54/1 -> b(54)/1, BodyDelay55/1
  b(54)/1 -> BodyLSum54/1
  BodyLSum54/1 -> BodyLSum55/2
  BodyDelay55/1 -> b(55)/1, BodyDelay56/1
  b(55)/1 -> BodyLSum55/1
  BodyLSum55/1 -> BodyLSum56/2
  BodyDelay56/1 -> b(56)/1, BodyDelay57/1
  b(56)/1 -> BodyLSum56/1
  BodyLSum56/1 -> BodyLSum57/2
  BodyDelay57/1 -> b(57)/1, BodyDelay58/1
  b(57)/1 -> BodyLSum57/1
  BodyLSum57/1 -> BodyLSum58/2
  BodyDelay58/1 -> b(58)/1, BodyDelay59/1
  b(58)/1 -> BodyLSum58/1
  BodyLSum58/1 -> BodyLSum59/2
  BodyDelay59/1 -> b(59)/1, BodyDelay60/1
  b(59)/1 -> BodyLSum59/1
  BodyLSum59/1 -> BodyLSum60/2
  BodyDelay60/1 -> b(60)/1, BodyDelay61/1
  b(60)/1 -> BodyLSum60/1
  BodyLSum60/1 -> BodyLSum61/2
  BodyDelay61/1 -> b(61)/1, BodyDelay62/1
  b(61)/1 -> BodyLSum61/1
  BodyLSum61/1 -> BodyLSum62/2
  BodyDelay62/1 -> b(62)/1, BodyDelay63/1
  b(62)/1 -> BodyLSum62/1
  BodyLSum62/1 -> BodyLSum63/2
  BodyDelay63/1 -> b(63)/1, BodyDelay64/1
  b(63)/1 -> BodyLSum63/1
  BodyLSum63/1 -> BodyLSum64/2
  BodyDelay64/1 -> b(64)/1, BodyDelay65/1
  b(64)/1 -> BodyLSum64/1
  BodyLSum64/1 -> BodyLSum65/2
  BodyDelay65/1 -> b(65)/1, BodyDelay66/1
  b(65)/1 -> BodyLSum65/1
  BodyLSum65/1 -> BodyLSum66/2
  BodyDelay66/1 -> b(66)/1, BodyDelay67/1
  b(66)/1 -> BodyLSum66/1
  BodyLSum66/1 -> BodyLSum67/2
  BodyDelay67/1 -> b(67)/1, BodyDelay68/1
  b(67)/1 -> BodyLSum67/1
  BodyLSum67/1 -> BodyLSum68/2
  BodyDelay68/1 -> b(68)/1, BodyDelay69/1
  b(68)/1 -> BodyLSum68/1
  BodyLSum68/1 -> BodyLSum69/2
  BodyDelay69/1 -> b(69)/1, BodyDelay70/1
  b(69)/1 -> BodyLSum69/1
  BodyLSum69/1 -> BodyLSum70/2
  BodyDelay70/1 -> b(70)/1, BodyDelay71/1
  b(70)/1 -> BodyLSum70/1
  BodyLSum70/1 -> BodyLSum71/2
  BodyDelay71/1 -> b(71)/1, BodyDelay72/1
  b(71)/1 -> BodyLSum71/1
  BodyLSum71/1 -> BodyLSum72/2
  BodyDelay72/1 -> b(72)/1, BodyDelay73/1
  b(72)/1 -> BodyLSum72/1
  BodyLSum72/1 -> BodyLSum73/2
  BodyDelay73/1 -> b(73)/1, BodyDelay74/1
  b(73)/1 -> BodyLSum73/1
  BodyLSum73/1 -> BodyLSum74/2
  BodyDelay74/1 -> b(74)/1, BodyDelay75/1
  b(74)/1 -> BodyLSum74/1
  BodyLSum74/1 -> BodyLSum75/2
  BodyDelay75/1 -> b(75)/1, BodyDelay76/1
  b(75)/1 -> BodyLSum75/1
  BodyLSum75/1 -> BodyLSum76/2
  BodyDelay76/1 -> b(76)/1, BodyDelay77/1
  b(76)/1 -> BodyLSum76/1
  BodyLSum76/1 -> BodyLSum77/2
  BodyDelay77/1 -> b(77)/1, BodyDelay78/1
  b(77)/1 -> BodyLSum77/1
  BodyLSum77/1 -> BodyLSum78/2
  BodyDelay78/1 -> b(78)/1, BodyDelay79/1
  b(78)/1 -> BodyLSum78/1
  BodyLSum78/1 -> BodyLSum79/2
  BodyDelay79/1 -> b(79)/1, BodyDelay80/1
  b(79)/1 -> BodyLSum79/1
  BodyLSum79/1 -> BodyLSum80/1
  BodyDelay80/1 -> b(80)/1
  b(80)/1 -> BodyLSum80/2
  BodyLSum80/1 -> ConvertOut/1
  ConvertOut/1 -> Output/1

== system Simulation1/Delta_Sigma_Modulator ==
  Baseband signal : Inport
  Eight_Order_Delta_Sigma_Modulator : Subsystem
  Fourth_Order_Delta_Sigma_Modulator_Simulation : Subsystem
  Second_Order_Delta_Sigma_Modulator_Simulation : Subsystem
  DAC_OUT1 : Outport
  DAC_OUT2 : Outport  Port=2
  DAC_OUT3 : Outport  Port=3
  wires:
  Second_Order_Delta_Sigma_Modulator_Simulation/1(Bitstream) -> DAC_OUT1/1  "Modulator output"
  Fourth_Order_Delta_Sigma_Modulator_Simulation/1(Bitstream) -> DAC_OUT2/1  "Modulator output"
  Eight_Order_Delta_Sigma_Modulator/1(Bitstream) -> DAC_OUT3/1  "Modulator output"
  Baseband signal/1 -> Eight_Order_Delta_Sigma_Modulator/1(Baseband signal), Fourth_Order_Delta_Sigma_Modulator_Simulation/1(Baseband Signal), Second_Order_Delta_Sigma_Modulator_Simulation/1(Baseband signal)

== system Simulation1/Delta_Sigma_Modulator1 ==
  Baseband signal : Inport
  Eight_Order_Delta_Sigma_Modulator : Subsystem
  Fourth_Order_Delta_Sigma_Modulator_Simulation : Subsystem
  Second_Order_Delta_Sigma_Modulator_Simulation : Subsystem
  DAC_OUT1 : Outport
  DAC_OUT2 : Outport  Port=2
  DAC_OUT3 : Outport  Port=3
  wires:
  Second_Order_Delta_Sigma_Modulator_Simulation/1(Bitstream) -> DAC_OUT1/1  "Modulator output"
  Fourth_Order_Delta_Sigma_Modulator_Simulation/1(Bitstream) -> DAC_OUT2/1  "Modulator output"
  Eight_Order_Delta_Sigma_Modulator/1(Bitstream) -> DAC_OUT3/1  "Modulator output"
  Baseband signal/1 -> Eight_Order_Delta_Sigma_Modulator/1(Baseband signal), Fourth_Order_Delta_Sigma_Modulator_Simulation/1(Baseband Signal), Second_Order_Delta_Sigma_Modulator_Simulation/1(Baseband signal)

== system Simulation1/Delta_Sigma_Modulator2 ==
  Baseband signal : Inport
  Eight_Order_Delta_Sigma_Modulator : Subsystem
  Fourth_Order_Delta_Sigma_Modulator_Simulation : Subsystem
  Second_Order_Delta_Sigma_Modulator_Simulation : Subsystem
  DAC_OUT1 : Outport
  DAC_OUT2 : Outport  Port=2
  DAC_OUT3 : Outport  Port=3
  wires:
  Second_Order_Delta_Sigma_Modulator_Simulation/1(Bitstream) -> DAC_OUT1/1  "Modulator output"
  Fourth_Order_Delta_Sigma_Modulator_Simulation/1(Bitstream) -> DAC_OUT2/1  "Modulator output"
  Eight_Order_Delta_Sigma_Modulator/1(Bitstream) -> DAC_OUT3/1  "Modulator output"
  Baseband signal/1 -> Eight_Order_Delta_Sigma_Modulator/1(Baseband signal), Fourth_Order_Delta_Sigma_Modulator_Simulation/1(Baseband Signal), Second_Order_Delta_Sigma_Modulator_Simulation/1(Baseband signal)

== system Simulation1/Halfband_1_61_44_Double_Precision ==
  Input : Inport
  InterpSys : Subsystem  Tag=FilterWizardInterpolatorCommutator
  bodygain1(2) : Gain  Gain=0.599649954166627031  ParamDataTypeStr=double  RndMeth=Nearest  SaturateOnIntegerOverflow=on  OutDataTypeStr=Inherit: Same as input
  bodygain1(3) : Gain  Gain=0.599649954166627031  ParamDataTypeStr=double  RndMeth=Nearest  SaturateOnIntegerOverflow=on  OutDataTypeStr=Inherit: Same as input
  bodygain1(4) : Gain  Gain=-0.122662452732889893  ParamDataTypeStr=double  RndMeth=Nearest  SaturateOnIntegerOverflow=on  OutDataTypeStr=Inherit: Same as input
  bodysum(1)2 : Sum  Inputs=++|  RndMeth=Nearest  SaturateOnIntegerOverflow=on  OutDataTypeStr=Inherit: Same as first input
  bodysum(1)3 : Sum  Inputs=++|  RndMeth=Nearest  SaturateOnIntegerOverflow=on  OutDataTypeStr=Inherit: Same as first input
  bodysum(1)4 : Sum  Inputs=++|  RndMeth=Nearest  SaturateOnIntegerOverflow=on  OutDataTypeStr=Inherit: Same as first input
  headgain1(1) : Gain  Gain=-0.122662452732889893  ParamDataTypeStr=double  RndMeth=Nearest  SaturateOnIntegerOverflow=on  OutDataTypeStr=Inherit: Same as input
  shareddelay2 : Delay  DelayLength=1  InitialCondition=0
  shareddelay3 : Delay  DelayLength=1  InitialCondition=0
  shareddelay4 : Delay  DelayLength=1  InitialCondition=0
  Output : Outport
  wires:
  headgain1(1)/1 -> bodysum(1)2/2
  Input/1 -> headgain1(1)/1, shareddelay2/1
  bodygain1(2)/1 -> bodysum(1)2/1
  bodysum(1)2/1 -> bodysum(1)3/2
  shareddelay2/1 -> bodygain1(2)/1, InterpSys/2(input2), shareddelay3/1
  bodygain1(3)/1 -> bodysum(1)3/1
  bodysum(1)3/1 -> bodysum(1)4/2
  shareddelay3/1 -> bodygain1(3)/1, shareddelay4/1
  bodygain1(4)/1 -> bodysum(1)4/1
  bodysum(1)4/1 -> InterpSys/1(input1)
  shareddelay4/1 -> bodygain1(4)/1
  InterpSys/1(output) -> Output/1
